simulink model "Dynamic_Control"  (R2015b)
settings: Solver=ode8  StartTime=0  StopTime=26  FixedStep=0.01  RelTol=1e-3
values from neighbouring files (symbols this model uses):
  Beta0 = pi    (= 3.14159265359)    [init.m]
  d = 0.15    [init.m]
  Kd = 8    [init.m]
  Kp = 8    [init.m]
  L = 0.13    [init.m]
  r = 0.1    [init.m]
  R = 2    [init.m]
  Theta0 = pi    (= 3.14159265359)    [init.m]
  wd = 0.5    [init.m]
  X0 = 2.3    [init.m]
  Y0 = 0    [init.m]
undefined symbols (not defined in the file): alpha
libraries: simulink x2
settings Model: Creator=GANESH  LastModifiedBy=GANESH

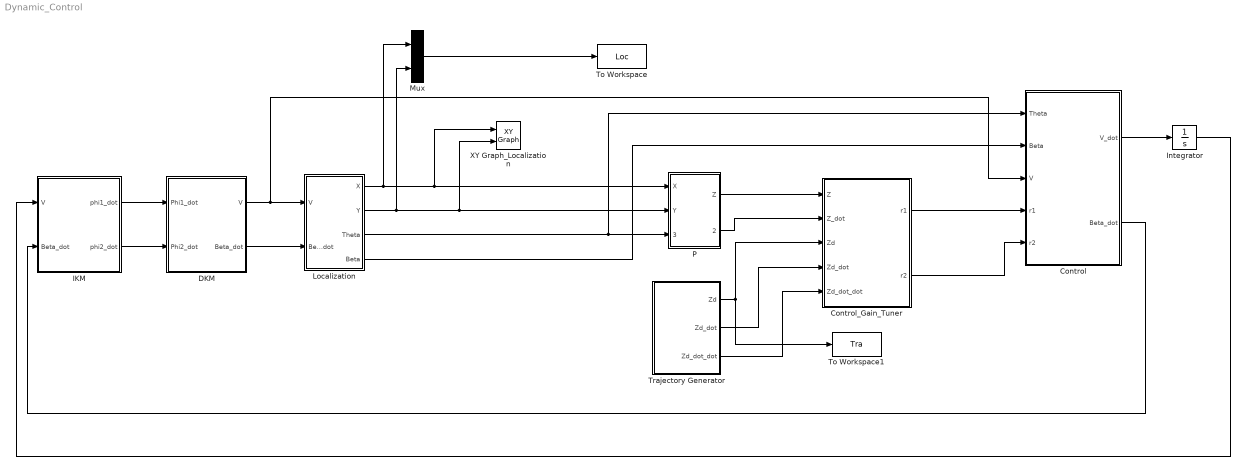
== system Dynamic_Control ==
  Control : Subsystem
  Control_Gain_Tuner : Subsystem
  DKM : Subsystem  mask{r=r}
      mask prompts: r "Radius of Wheel"
  IKM : Subsystem  mask{r=(1+alpha)*r}
      mask prompts: r "Radius of Wheel"
  Integrator : Integrator  InitialCondition=0.1
  Localization : Subsystem  mask{Parameter1=L}
      mask prompts: Parameter1 "Half of WheelBase"
  Mux : Mux  Inputs=2
  P : Subsystem  mask{d=0}
      mask prompts: d "Distance of point P"
  To Workspace : ToWorkspace  VariableName=Loc  SaveFormat=Timeseries  SampleTime=-1
  To Workspace1 : ToWorkspace  VariableName=Tra  SaveFormat=Timeseries  SampleTime=-1
  Trajectory Generator : Subsystem  mask{R=R}
      mask prompts: R "Radius of Trajectory"
  XY Graph_Localization : simulink/Sinks/XY Graph  xmin=-5  xmax=5  ymin=-5  ymax=5  st=-1
  wires:
  Localization/1(X) -> Mux/1, XY Graph_Localization/1, P/1(X)
  Localization/2(Y) -> Mux/2, XY Graph_Localization/2, P/2(Y)
  Localization/3(Theta) -> Control/1(Theta), P/3(Theta)
  Localization/4(Beta) -> Control/2(Beta)
  IKM/2(phi2_dot) -> DKM/2(Phi2_dot)
  P/1(Z) -> Control_Gain_Tuner/1(Z)
  Trajectory Generator/1(Zd) -> Control_Gain_Tuner/3(Zd), To Workspace1/1
  IKM/1(phi1_dot) -> DKM/1(Phi1_dot)
  DKM/2(Beta_dot) -> Localization/2(Beta_dot)
  Trajectory Generator/2(Zd_dot) -> Control_Gain_Tuner/4(Zd_dot)
  Trajectory Generator/3(Zd_dot_dot) -> Control_Gain_Tuner/5(Zd_dot_dot)
  P/2(Z_dot) -> Control_Gain_Tuner/2(Z_dot)
  Control/1(V_dot) -> Integrator/1
  Control/2(Beta_dot) -> IKM/2(Beta_dot)
  Integrator/1 -> IKM/1(V)
  Control_Gain_Tuner/1(r1) -> Control/4(r1)
  Control_Gain_Tuner/2(r2) -> Control/5(r2)
  DKM/1(V) -> Control/3(V), Localization/1(V)
  Mux/1 -> To Workspace/1

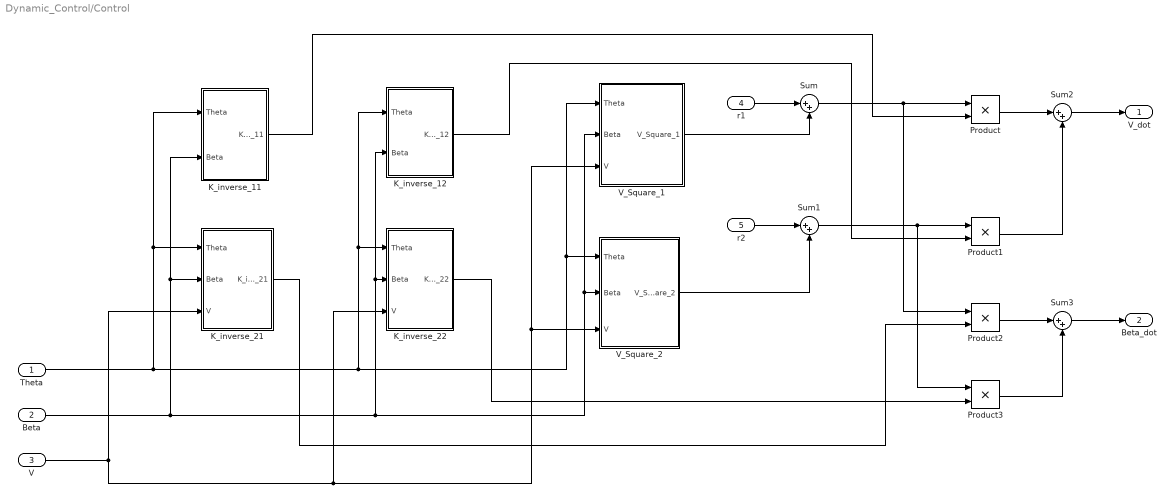
== system Dynamic_Control/Control ==
  Theta : Inport
  Beta : Inport  Port=2
  V : Inport  Port=3
  r1 : Inport  Port=4
  r2 : Inport  Port=5
  K_inverse_11 : Subsystem
  K_inverse_12 : Subsystem
  K_inverse_21 : Subsystem
  K_inverse_22 : Subsystem
  Product{,1..3} (4 alike) : Product
  Sum{,1..3} (4 alike) : Sum  Inputs=|++
  V_Square_1 : Subsystem
  V_Square_2 : Subsystem
  V_dot : Outport
  Beta_dot : Outport  Port=2
  wires:
  Beta/1 -> K_inverse_11/2(Beta), K_inverse_21/2(Beta), K_inverse_12/2(Beta), K_inverse_22/2(Beta), V_Square_1/2(Beta), V_Square_2/2(Beta)
  Theta/1 -> K_inverse_11/1(Theta), K_inverse_21/1(Theta), K_inverse_12/1(Theta), K_inverse_22/1(Theta), V_Square_2/1(Theta), V_Square_1/1(Theta)
  V/1 -> K_inverse_22/3(V), V_Square_2/3(V), V_Square_1/3(V), K_inverse_21/3(V)
  r1/1 -> Sum/1
  V_Square_1/1(V_Square_1) -> Sum/2
  r2/1 -> Sum1/1
  V_Square_2/1(V_Square_2) -> Sum1/2
  Sum/1 -> Product2/1, Product/1
  K_inverse_11/1(K_inverse_11) -> Product/2
  Sum1/1 -> Product3/1, Product1/1
  K_inverse_12/1(K_inverse_12) -> Product1/2
  Product/1 -> Sum2/1
  Product1/1 -> Sum2/2
  Sum2/1 -> V_dot/1
  K_inverse_21/1(K_inverse_21) -> Product2/2
  K_inverse_22/1(K_inverse_22) -> Product3/2
  Product2/1 -> Sum3/1
  Product3/1 -> Sum3/2
  Sum3/1 -> Beta_dot/1

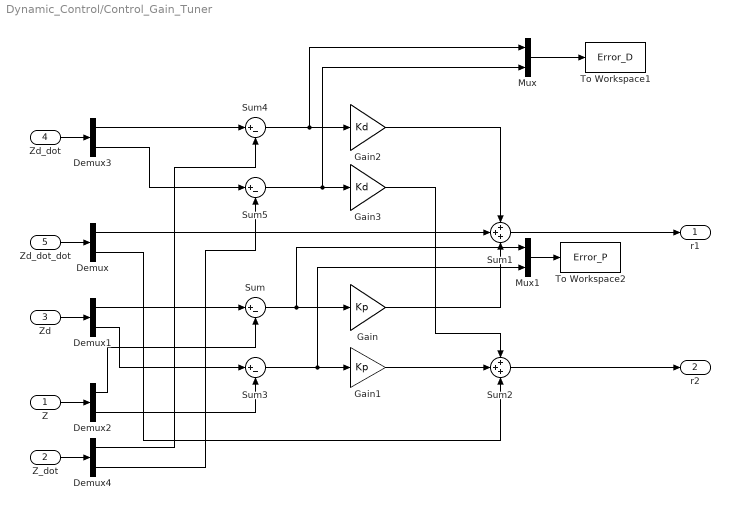
== system Dynamic_Control/Control_Gain_Tuner ==
  Z : Inport
  Z_dot : Inport  Port=2
  Zd : Inport  Port=3
  Zd_dot : Inport  Port=4
  Zd_dot_dot : Inport  Port=5
  Demux{,1..4} (5 alike) : Demux  Outputs=2
  Gain : Gain  Gain=Kp
  Gain1 : Gain  Gain=Kp
  Gain2 : Gain  Gain=Kd
  Gain3 : Gain  Gain=Kd
  Mux : Mux  Inputs=2
  Mux1 : Mux  Inputs=2
  Sum{,3..5} (4 alike) : Sum  Inputs=|+-
  Sum1 : Sum  Inputs=+++
  Sum2 : Sum  Inputs=+++
  To Workspace1 : ToWorkspace  VariableName=Error_D  SaveFormat=Timeseries  SampleTime=-1
  To Workspace2 : ToWorkspace  VariableName=Error_P  SaveFormat=Timeseries  SampleTime=-1
  r1 : Outport
  r2 : Outport  Port=2
  wires:
  Demux2/2 -> Sum3/2
  Demux1/1 -> Sum/1
  Gain/1 -> Sum1/3
  Demux2/1 -> Sum/2
  Zd_dot_dot/1 -> Demux/1
  Gain1/1 -> Sum2/2
  Demux/1 -> Sum1/2
  Sum3/1 -> Mux1/2, Gain1/1
  Demux1/2 -> Sum3/1
  Sum1/1 -> r1/1
  Zd/1 -> Demux1/1
  Demux/2 -> Sum2/3
  Sum2/1 -> r2/1
  Sum/1 -> Mux1/1, Gain/1
  Z/1 -> Demux2/1
  Zd_dot/1 -> Demux3/1
  Sum4/1 -> Mux/1, Gain2/1
  Demux3/1 -> Sum4/1
  Gain2/1 -> Sum1/1
  Z_dot/1 -> Demux4/1
  Demux4/1 -> Sum4/2
  Sum5/1 -> Mux/2, Gain3/1
  Demux3/2 -> Sum5/1
  Demux4/2 -> Sum5/2
  Gain3/1 -> Sum2/1
  Mux/1 -> To Workspace1/1
  Mux1/1 -> To Workspace2/1

== system Dynamic_Control/DKM ==
  Phi1_dot : Inport
  Phi2_dot : Inport  Port=2
  Constant : Constant  Value=r
  Product2 : Product
  V : Outport
  Beta_dot : Outport  Port=2
  wires:
  Phi1_dot/1 -> Product2/2
  Phi2_dot/1 -> Beta_dot/1
  Constant/1 -> Product2/1
  Product2/1 -> V/1

== system Dynamic_Control/IKM ==
  V : Inport
  Beta_dot : Inport  Port=2
  Constant1 : Constant  Value=r
  Divide1 : Product  Inputs=*/
  phi1_dot : Outport
  phi2_dot : Outport  Port=2
  wires:
  V/1 -> Divide1/1
  Beta_dot/1 -> phi2_dot/1
  Constant1/1 -> Divide1/2
  Divide1/1 -> phi1_dot/1

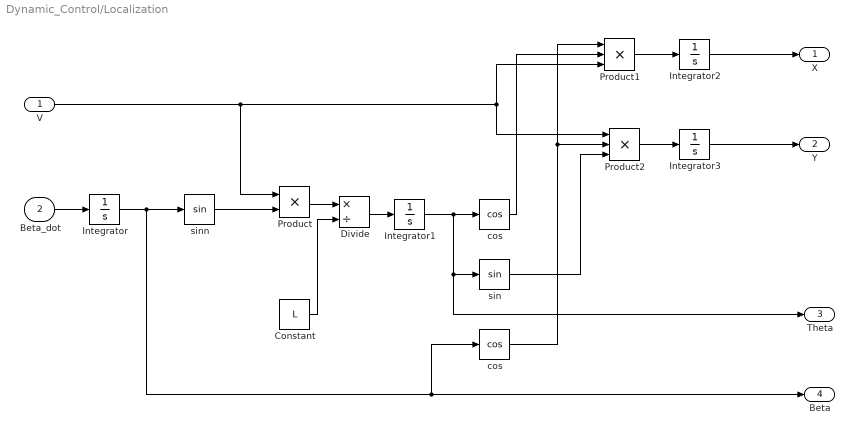
== system Dynamic_Control/Localization ==
  V : Inport
  Beta_dot : Inport  Port=2
  Constant : Constant  Value=L
  Divide : Product  Inputs=*/
  Integrator : Integrator  InitialCondition=Beta0
  Integrator1 : Integrator  InitialCondition=Theta0
  Integrator2 : Integrator  InitialCondition=X0
  Integrator3 : Integrator  InitialCondition=Y0
  Product : Product
  Product1 : Product  Inputs=3
  Product2 : Product  Inputs=3
  cos : Trigonometry  Operator=cos
  "cos " : Trigonometry  Operator=cos
  sin : Trigonometry
  sinn : Trigonometry
  X : Outport
  Y : Outport  Port=2
  Theta : Outport  Port=3
  Beta : Outport  Port=4
  wires:
  Integrator1/1 -> Theta/1, sin/1, "cos "/1
  Product2/1 -> Integrator3/1
  Integrator3/1 -> Y/1
  V/1 -> Product1/3, Product2/1, Product/1
  Product/1 -> Divide/1
  Integrator/1 -> sinn/1, cos/1, Beta/1
  Product1/1 -> Integrator2/1
  Integrator2/1 -> X/1
  Divide/1 -> Integrator1/1
  Beta_dot/1 -> Integrator/1
  sinn/1 -> Product/2
  Constant/1 -> Divide/2
  cos/1 -> Product1/1, Product2/2
  "cos "/1 -> Product1/2
  sin/1 -> Product2/3

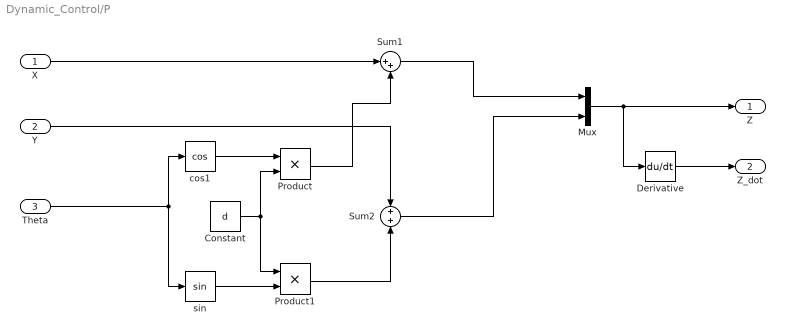
== system Dynamic_Control/P ==
  X : Inport
  Y : Inport  Port=2
  Theta : Inport  Port=3
  Constant : Constant  Value=d
  Derivative : Derivative
  Mux : Mux  Inputs=2
  Product : Product
  Product1 : Product
  Sum1 : Sum  Inputs=|++
  Sum2 : Sum
  cos1 : Trigonometry  Operator=cos
  sin : Trigonometry
  Z : Outport
  Z_dot : Outport  Port=2
  wires:
  Mux/1 -> Derivative/1, Z/1
  Sum1/1 -> Mux/1
  X/1 -> Sum1/1
  Y/1 -> Sum2/1
  Theta/1 -> sin/1, cos1/1
  Sum2/1 -> Mux/2
  sin/1 -> Product1/2
  Product1/1 -> Sum2/2
  cos1/1 -> Product/1
  Constant/1 -> Product1/1, Product/2
  Derivative/1 -> Z_dot/1
  Product/1 -> Sum1/2

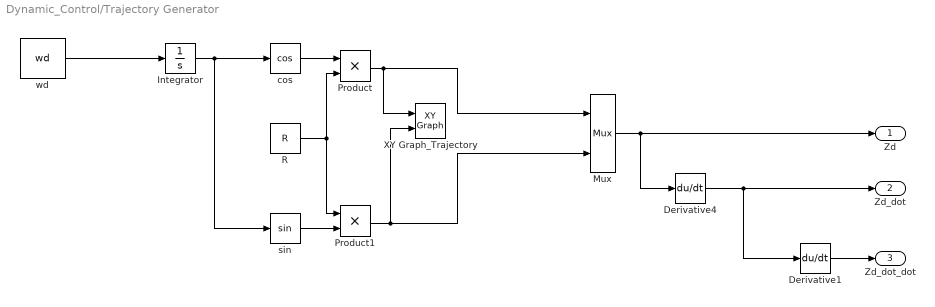
== system Dynamic_Control/Trajectory Generator ==
  Derivative1 : Derivative
  Derivative4 : Derivative
  Integrator : Integrator
  Mux : Mux  Inputs=2
  Product : Product
  Product1 : Product
  R : Constant  Value=R
  XY Graph_Trajectory : simulink/Sinks/XY Graph  xmin=-5  xmax=5  ymin=-5  ymax=5  st=-1
  cos : Trigonometry  Operator=cos
  sin : Trigonometry
  wd : Constant  Value=wd
  Zd : Outport
  Zd_dot : Outport  Port=2
  Zd_dot_dot : Outport  Port=3
  wires:
  Mux/1 -> Derivative4/1, Zd/1
  R/1 -> Product1/1, Product/2
  Product1/1 -> XY Graph_Trajectory/2, Mux/2
  wd/1 -> Integrator/1
  cos/1 -> Product/1
  Integrator/1 -> sin/1, cos/1
  sin/1 -> Product1/2
  Product/1 -> XY Graph_Trajectory/1, Mux/1
  Derivative4/1 -> Derivative1/1, Zd_dot/1
  Derivative1/1 -> Zd_dot_dot/1

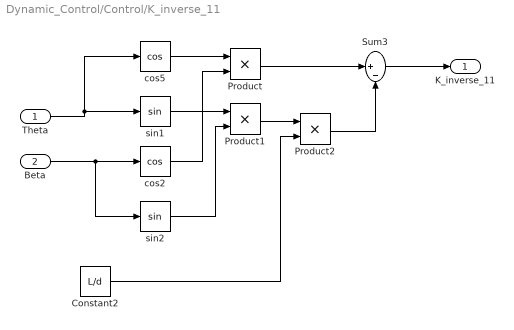
== system Dynamic_Control/Control/K_inverse_11 ==
  Theta : Inport
  Beta : Inport  Port=2
  Constant2 : Constant  Value=L/d
  Product : Product
  Product1 : Product
  Product2 : Product
  Sum3 : Sum  Inputs=|+-
  cos2 : Trigonometry  Operator=cos
  cos5 : Trigonometry  Operator=cos
  sin1 : Trigonometry
  sin2 : Trigonometry
  K_inverse_11 : Outport
  wires:
  Theta/1 -> sin1/1, cos5/1
  Beta/1 -> sin2/1, cos2/1
  cos5/1 -> Product/1
  cos2/1 -> Product/2
  sin1/1 -> Product1/1
  sin2/1 -> Product1/2
  Product1/1 -> Product2/1
  Constant2/1 -> Product2/2
  Product/1 -> Sum3/1
  Product2/1 -> Sum3/2
  Sum3/1 -> K_inverse_11/1

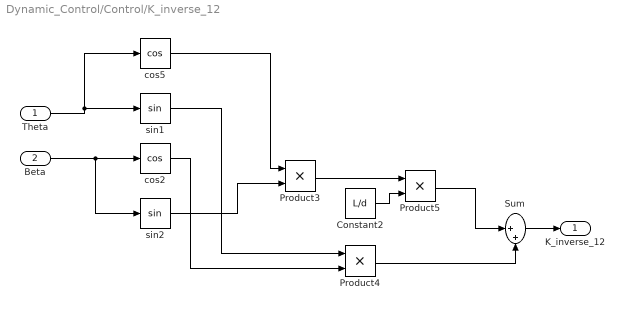
== system Dynamic_Control/Control/K_inverse_12 ==
  Theta : Inport
  Beta : Inport  Port=2
  Constant2 : Constant  Value=L/d
  Product3 : Product
  Product4 : Product
  Product5 : Product
  Sum : Sum  Inputs=|++
  cos2 : Trigonometry  Operator=cos
  cos5 : Trigonometry  Operator=cos
  sin1 : Trigonometry
  sin2 : Trigonometry
  K_inverse_12 : Outport
  wires:
  Theta/1 -> sin1/1, cos5/1
  Beta/1 -> sin2/1, cos2/1
  cos5/1 -> Product3/1
  cos2/1 -> Product4/2
  sin1/1 -> Product4/1
  sin2/1 -> Product3/2
  Constant2/1 -> Product5/2
  Product3/1 -> Product5/1
  Product5/1 -> Sum/1
  Product4/1 -> Sum/2
  Sum/1 -> K_inverse_12/1

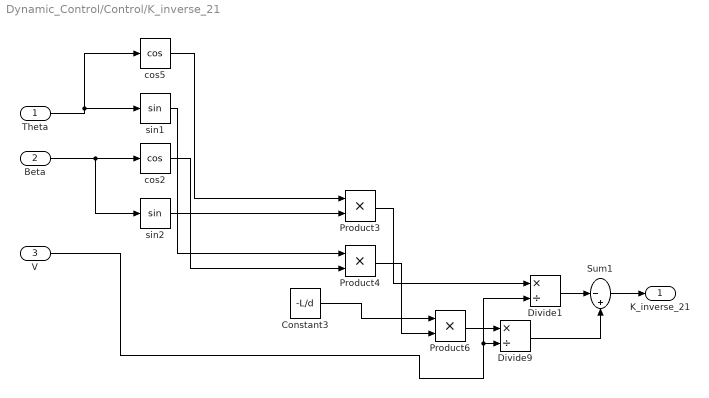
== system Dynamic_Control/Control/K_inverse_21 ==
  Theta : Inport
  Beta : Inport  Port=2
  V : Inport  Port=3
  Constant3 : Constant  Value=-L/d
  Divide1 : Product  Inputs=*/
  Divide9 : Product  Inputs=*/
  Product3 : Product
  Product4 : Product
  Product6 : Product
  Sum1 : Sum  Inputs=|-+
  cos2 : Trigonometry  Operator=cos
  cos5 : Trigonometry  Operator=cos
  sin1 : Trigonometry
  sin2 : Trigonometry
  K_inverse_21 : Outport
  wires:
  Theta/1 -> sin1/1, cos5/1
  Beta/1 -> sin2/1, cos2/1
  cos5/1 -> Product3/1
  cos2/1 -> Product4/2
  sin1/1 -> Product4/1
  sin2/1 -> Product3/2
  Product3/1 -> Divide1/1
  Product4/1 -> Product6/2
  Constant3/1 -> Product6/1
  Product6/1 -> Divide9/1
  V/1 -> Divide1/2, Divide9/2
  Divide1/1 -> Sum1/1
  Sum1/1 -> K_inverse_21/1
  Divide9/1 -> Sum1/2

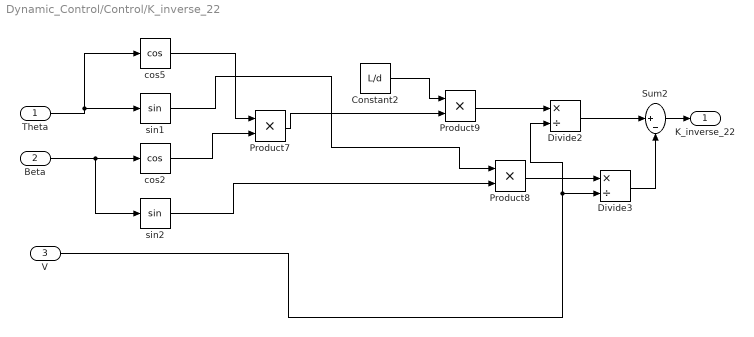
== system Dynamic_Control/Control/K_inverse_22 ==
  Theta : Inport
  Beta : Inport  Port=2
  V : Inport  Port=3
  Constant2 : Constant  Value=L/d
  Divide2 : Product  Inputs=*/
  Divide3 : Product  Inputs=*/
  Product7 : Product
  Product8 : Product
  Product9 : Product
  Sum2 : Sum  Inputs=|+-
  cos2 : Trigonometry  Operator=cos
  cos5 : Trigonometry  Operator=cos
  sin1 : Trigonometry
  sin2 : Trigonometry
  K_inverse_22 : Outport
  wires:
  Theta/1 -> sin1/1, cos5/1
  Beta/1 -> sin2/1, cos2/1
  cos5/1 -> Product7/1
  cos2/1 -> Product7/2
  sin1/1 -> Product8/1
  sin2/1 -> Product8/2
  V/1 -> Divide2/2, Divide3/2
  Product7/1 -> Product9/2
  Product9/1 -> Divide2/1
  Divide2/1 -> Sum2/1
  Product8/1 -> Divide3/1
  Divide3/1 -> Sum2/2
  Sum2/1 -> K_inverse_22/1
  Constant2/1 -> Product9/1

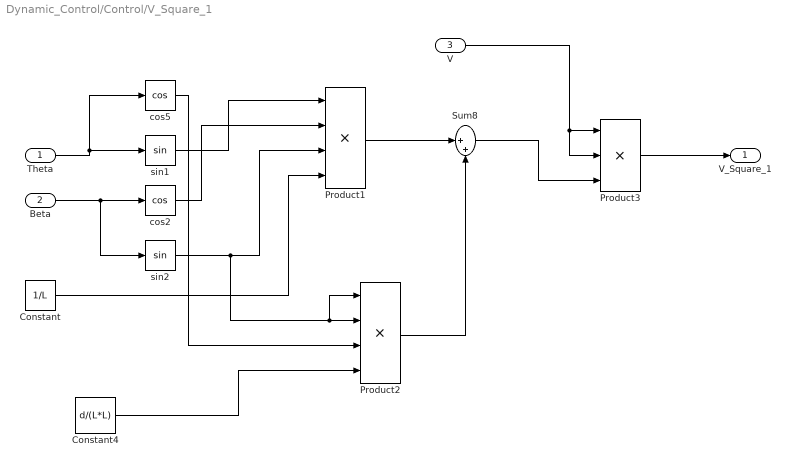
== system Dynamic_Control/Control/V_Square_1 ==
  Theta : Inport
  Beta : Inport  Port=2
  V : Inport  Port=3
  Constant : Constant  Value=1/L
  Constant4 : Constant  Value=d/(L*L)
  Product1 : Product  Inputs=4
  Product2 : Product  Inputs=4
  Product3 : Product  Inputs=3
  Sum8 : Sum  Inputs=|++
  cos2 : Trigonometry  Operator=cos
  cos5 : Trigonometry  Operator=cos
  sin1 : Trigonometry
  sin2 : Trigonometry
  V_Square_1 : Outport
  wires:
  Theta/1 -> sin1/1, cos5/1
  Beta/1 -> sin2/1, cos2/1
  V/1 -> Product3/1, Product3/2
  sin1/1 -> Product1/1
  cos2/1 -> Product1/2
  sin2/1 -> Product2/1, Product2/2, Product1/3
  Constant/1 -> Product1/4
  Product1/1 -> Sum8/1
  Constant4/1 -> Product2/4
  cos5/1 -> Product2/3
  Product2/1 -> Sum8/2
  Sum8/1 -> Product3/3
  Product3/1 -> V_Square_1/1

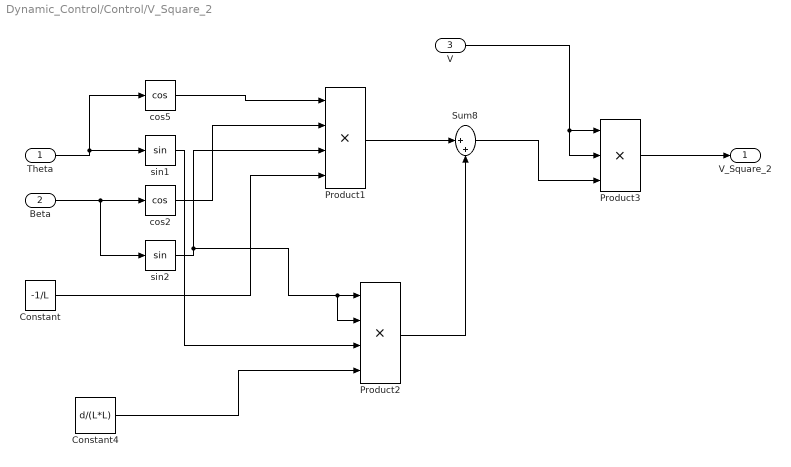
== system Dynamic_Control/Control/V_Square_2 ==
  Theta : Inport
  Beta : Inport  Port=2
  V : Inport  Port=3
  Constant : Constant  Value=-1/L
  Constant4 : Constant  Value=d/(L*L)
  Product1 : Product  Inputs=4
  Product2 : Product  Inputs=4
  Product3 : Product  Inputs=3
  Sum8 : Sum  Inputs=|++
  cos2 : Trigonometry  Operator=cos
  cos5 : Trigonometry  Operator=cos
  sin1 : Trigonometry
  sin2 : Trigonometry
  V_Square_2 : Outport
  wires:
  Theta/1 -> sin1/1, cos5/1
  Beta/1 -> sin2/1, cos2/1
  V/1 -> Product3/1, Product3/2
  Product1/1 -> Sum8/1
  Product2/1 -> Sum8/2
  Sum8/1 -> Product3/3
  Product3/1 -> V_Square_2/1
  Constant/1 -> Product1/4
  cos5/1 -> Product1/1
  cos2/1 -> Product1/2
  sin2/1 -> Product1/3, Product2/2, Product2/1
  Constant4/1 -> Product2/4
  sin1/1 -> Product2/3
